simulink model "Parqueadero_2"  (R2020b)
settings: Solver=VariableStepAuto  StartTime=0.0  StopTime=20  RelTol=1e-3
settings Model: Creator=mateo  LastModifiedBy=mateo

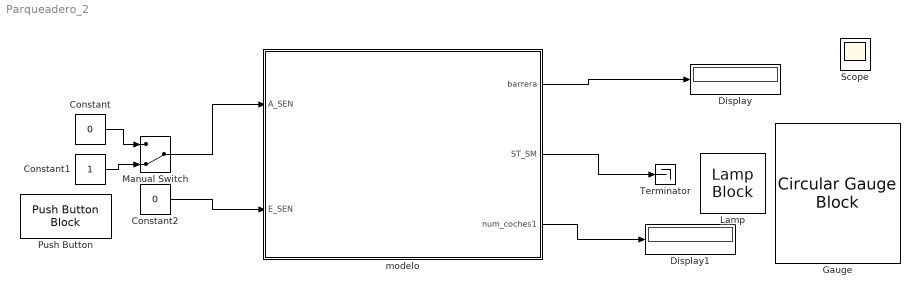
== system Parqueadero_2 ==
  Constant : Constant  Value=0
  Constant1 : Constant
  Constant2 : Constant  Value=0
  Display : Display
  Display1 : Display
  Gauge : CircularGaugeBlock  ScaleMax=10
  Lamp : LampBlock
  Manual Switch : ManualSwitch  CurrentSetting=0
  Push Button : PushButtonBlock
  Scope : Scope  NumInputPorts=3
  Terminator : Terminator
  modelo : Subsystem
  wires:
  Constant/1 -> Manual Switch/1
  Constant1/1 -> Manual Switch/2
  Manual Switch/1 -> modelo/1(A_SEN)
  Constant2/1 -> modelo/2(E_SEN)
  modelo/1(barrera) -> Display/1
  modelo/2(ST_SM) -> Terminator/1
  modelo/3(num_coches1) -> Display1/1

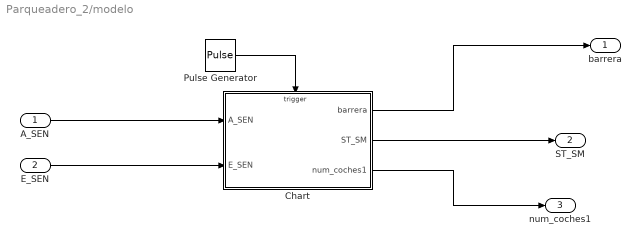
== system Parqueadero_2/modelo ==
  A_SEN : Inport
  E_SEN : Inport  Port=2
  Chart : Stateflow chart  TreatAsAtomicUnit=on
  Pulse Generator : DiscretePulseGenerator  PulseType=Time based  Period=0.5  PulseWidth=50
  barrera : Outport
  ST_SM : Outport  Port=2
  num_coches1 : Outport  Port=3
  wires:
  Pulse Generator/1 -> Chart/Trigger
  A_SEN/1 -> Chart/1(A_SEN)
  E_SEN/1 -> Chart/2(E_SEN)
  Chart/2(ST_SM) -> ST_SM/1
  Chart/1(barrera) -> barrera/1
  Chart/3(num_coches1) -> num_coches1/1

== stateflow chart Parqueadero_2/modelo/Chart ==
  state ESTADO_LIBRE
    state ENTRA_COCHE
      entry:
      barrera=1;
      num_coches=num_coches +1;
      num_coches1=num_coches;
    state ENTRA_COCHE_2
      entry:
      barrera=0;
    state PASO_OCUPADO
      entry:
      evento_ON_OFF=0;
      ST_SM=0;
    state INICIO
      entry:
      barrera=0;
    state SALE_COCHE
      entry:
      num_coches=num_coches -1;
      num_coches1=num_coches;
    ENTRA_COCHE_2 -> ESTADO_LIBRE.INICIO [order 2]
    (default) -> ESTADO_LIBRE.INICIO
    ESTADO_LIBRE.INICIO -> ENTRA_COCHE [order 1] : [A_SEN==1]
    ENTRA_COCHE_2 -> PASO_OCUPADO [order 1] : [num_coches==10]
    ENTRA_COCHE -> ENTRA_COCHE_2 : [A_SEN==0]
    SALE_COCHE -> ESTADO_LIBRE.INICIO : [E_SEN==0]
    ESTADO_LIBRE.INICIO -> SALE_COCHE [order 2] : [E_SEN==1]
  state ESTADO_OCUPADO
    state RESTA_COCHES
      entry:
      num_coches=num_coches-1;
      num_coches1=num_coches;
    state INICIO
      entry:
      barrera=0;
    state PASAR_LIBRE
      entry:
      evento_ON_OFF=1;
      ST_SM=1;
    (default) -> ESTADO_OCUPADO.INICIO
    ESTADO_OCUPADO.INICIO -> RESTA_COCHES : [E_SEN==1]
    RESTA_COCHES -> PASAR_LIBRE : [E_SEN==0]
  ESTADO_LIBRE -> ESTADO_OCUPADO : [evento_ON_OFF==0]
  (default) -> ESTADO_LIBRE
  ESTADO_OCUPADO -> ESTADO_LIBRE : [evento_ON_OFF==1]
  data: A_SEN input; E_SEN input; barrera output =0; ST_SM output =1; num_coches local =0; num_coches1 output =0; evento_ON_OFF local =1
  events: CLOCK input EITHER_EDGE_EVENT
